simulink model "dynamics"  (R2016a)
settings: Solver=ode45  StartTime=0.0  StopTime=20  RelTol=1e-3
values from neighbouring files (symbols this model uses):
  Jred = Jr+((Js+((m*p^2)/(4*pi^2)))/g^2)    [dynamicsoptimizing.m]    (also in gsimulate.m)
  p = 4*10^-3    (= 0.004)    [dynamicsoptimizing.m]    (also in gsimulate.m)
  Tmax = 5    [dynamicsoptimizing.m]    (also in gsimulate.m)
  wmax = 2*pi*(nmax/60)    (= 628.318530718)    [dynamicsoptimizing.m]    (also in gsimulate.m)
undefined symbols (not defined in the file or in its folder): g
libraries: simulink x1
settings Model: Creator=viitalr1  LastModifiedBy=tlantela
settings DataIOCC: LimitDataPoints=on  SaveFormat=Array
settings HardwareCC: ProdBitPerPointer=32  ProdLargestAtomicFloat=None  ProdIntDivRoundTo=Undefined  ProdEndianess=Unspecified  ProdWordSize=32  ProdHWDeviceType=32-bit Generic
settings ModelReferenceCC: PropagateSignalLabelsOutOfModel=off
settings ConfigComp: CovModelRefEnable=Off

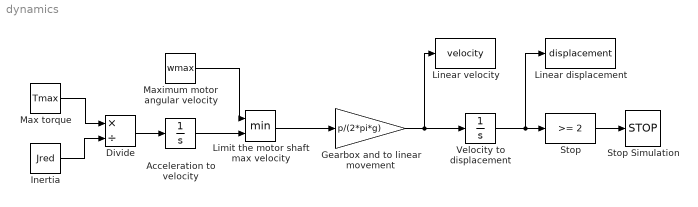
== system dynamics ==
  Acceleration to velocity : Integrator
  Divide : Product  Inputs=*/
  Gearbox and to linear movement : Gain  Gain=p/(2*pi*g)
  Inertia : Constant  Value=Jred
  Limit the motor shaft max velocity : MinMax  Inputs=2
  Linear displacement : ToWorkspace  VariableName=displacement  SaveFormat=Timeseries  SampleTime=-1
  Linear velocity : ToWorkspace  VariableName=velocity  SaveFormat=Timeseries  SampleTime=-1
  "Max torque " : Constant  Value=Tmax
  Maximum motor angular velocity : Constant  Value=wmax
  Stop : simulink/Logic and Bit Operations/Compare To Constant  relop=>=  const=2  OutDataTypeStr=boolean  ZeroCross=off
  Stop Simulation : Stop
  Velocity to displacement : Integrator
  wires:
  "Max torque "/1 -> Divide/1
  Inertia/1 -> Divide/2
  Maximum motor angular velocity/1 -> Limit the motor shaft max velocity/1
  Velocity to displacement/1 -> Linear displacement/1, Stop/1
  Stop/1 -> Stop Simulation/1
  Gearbox and to linear movement/1 -> Linear velocity/1, Velocity to displacement/1
  Acceleration to velocity/1 -> Limit the motor shaft max velocity/2
  Limit the motor shaft max velocity/1 -> Gearbox and to linear movement/1
  Divide/1 -> Acceleration to velocity/1
